simulink model "step_responses"  (R2023b)
settings: Solver=VariableStepAuto  StartTime=0.0  StopTime=10.0  RelTol=1e-3
values from neighbouring files (symbols this model uses):
  den = [1,5,8]    [FinalAlgorithm.m]
  dendi = zeros(1,n+1)    [FinalAlgorithm.m]
  num = 1    [FinalAlgorithm.m]
  numdi = zeros(1,n)    [FinalAlgorithm.m]
  ts = 1e-1    (= 0.1)    [FinalAlgorithm.m]
settings Model: Creator=AdrianCortez  LastModifiedBy=AdrianCortez

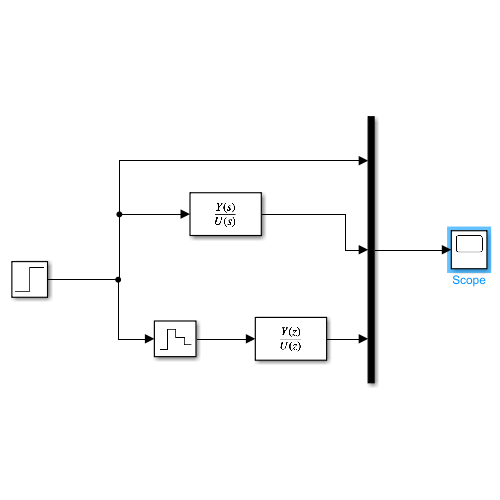
[thumbnail: Simulink's stored preview of the top-level diagram]
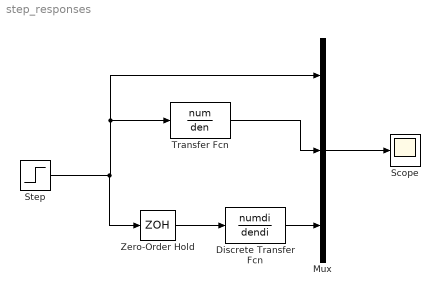
== system step_responses ==
  Discrete Transfer Fcn : DiscreteTransferFcn  Numerator=numdi  Denominator=dendi
  Mux : Mux  Inputs=3
  Scope : Scope
  Step : Step  SampleTime=0
  Transfer Fcn : TransferFcn  Numerator=num  Denominator=den
  Zero-Order Hold : ZeroOrderHold  SampleTime=ts
  wires:
  Step/1 -> Zero-Order Hold/1, Mux/1, Transfer Fcn/1
  Transfer Fcn/1 -> Mux/2
  Discrete Transfer Fcn/1 -> Mux/3
  Mux/1 -> Scope/1
  Zero-Order Hold/1 -> Discrete Transfer Fcn/1
